simulink model "Reactor_PDE_R2013a"  (R2013a)
settings: Solver=ode45  StartTime=0.0  StopTime=double(Tsim)  FixedStep=double(grampc.param.dt)  RelTol=1e-3
values from neighbouring files (symbols this model uses):
  grampc = grampc_update_struct_grampc(grampc,user)    [initData.m]    (also in startMPC.m = CmexFiles.grampc_setparam_Cmex(grampc,'x0',vec.x(:,i)))
settings Model: Creator=kaepernick  LastModifiedBy=koy47
settings OptimizationCC: ExpressionDepthLimit=2147483647
settings DebuggingCC: FrameProcessingCompatibilityMsg=error
settings GRTTargetCC: CodeReplacementLibrary=C89/C90 (ANSI)

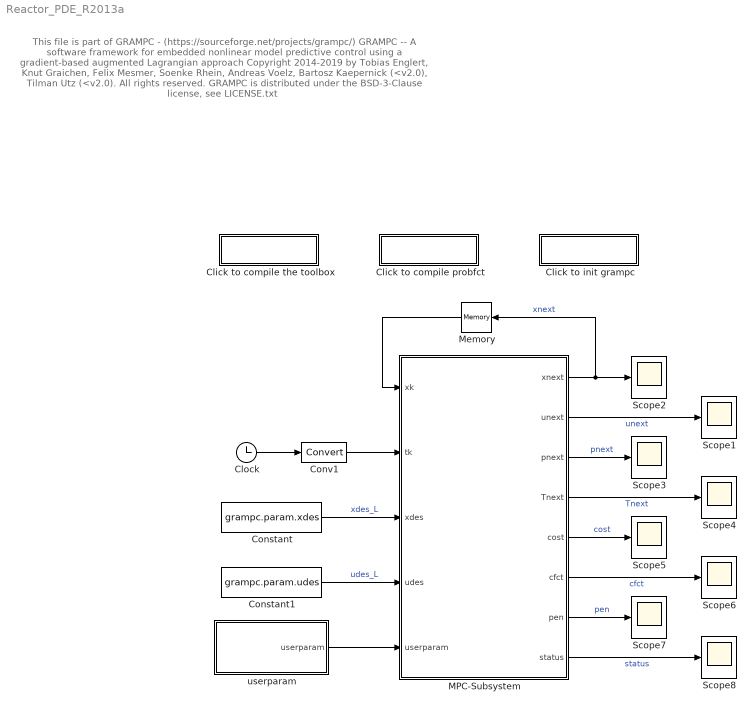
== system Reactor_PDE_R2013a ==
  note: This file is part of GRAMPC - (https://sourceforge.net/projects/grampc/)
      |
      | GRAMPC -- A software framework for embedded nonlinear model predictive
      | control using a gradient-based augmented Lagrangian approach
      |
      | Copyright 2014-2019 by Tobias Englert, Knut Graichen, Felix Mesmer,
      | Soenke Rhein, Andreas Voelz, Bartosz Kaepernick (<v2.0), Tilman Utz (<v2.0).
      | All rights reserved.
      |
      | GRAMPC is distributed under the BSD-3-Clause license, see LICENSE.txt
  Click to compile probfct : Subsystem
      settings: OpenFcn=|
      | cd(fileparts(which(gcs)))
      | grampc_path = '../../';
      | addpath([grampc_path 'matlab/mfiles']);
      | grampc_make_probfct(grampc_path,'probfct_REACTOR_PDE.c','clean');
  Click to compile the toolbox : Subsystem
      settings: OpenFcn=|
      | cd(fileparts(which(gcs)))
      | curdir = cd;
      | cd('../../matlab')
      | make clean
      | cd(curdir)
  Click to init grampc : Subsystem
      settings: OpenFcn=|
      | cd(fileparts(which(gcs)))
      | grampc_path = '../../';
      | addpath([grampc_path 'matlab/mfiles']);
      | [grampc,Tsim,grampc_sdata] = initData;
  Clock : Clock
  Constant : Constant  Value=grampc.param.xdes
  Constant1 : Constant  Value=grampc.param.udes
  Conv1 : DataTypeConversion
  MPC-Subsystem : Subsystem  TreatAsAtomicUnit=on  SystemSampleTime=double(grampc.param.dt)
  Memory : Memory  X0=grampc.param.x0
  Scope{1..8} (8 alike) : Scope
      Scope1 settings: TimeRange=auto  MaxDataPoints=5000  SaveToWorkspace=off  YMin=-2.5  YMax=2.5  SampleTime=-1
      Scope2 settings: TimeRange=auto  MaxDataPoints=5000  SaveToWorkspace=off  SaveName=ScopeData2  YMin=0.66111  YMax=2.14906  SampleTime=-1
      Scope3 settings: TimeRange=auto  MaxDataPoints=5000  SaveToWorkspace=off  SaveName=ScopeData3  YMin=-1.00000  YMax=1.00000  SampleTime=-1
      Scope4 settings: TimeRange=auto  MaxDataPoints=5000  SaveToWorkspace=off  SaveName=ScopeData4  YMin=0.5  YMax=2.5  SampleTime=-1
      Scope5 settings: TimeRange=auto  MaxDataPoints=5000  SaveToWorkspace=off  SaveName=ScopeData5  YMin=-0.1279  YMax=0.27397  SampleTime=-1
      Scope6 settings: TimeRange=auto  MaxDataPoints=5000  SaveToWorkspace=off  SaveName=ScopeData6  YMin=-0.15393  YMax=1.38537  SampleTime=-1
      Scope7 settings: TimeRange=auto  MaxDataPoints=5000  SaveToWorkspace=off  SaveName=ScopeData7  YMin=-28.95426  YMax=270.07514  SampleTime=-1
      Scope8 settings: TimeRange=auto  MaxDataPoints=5000  SaveToWorkspace=off  SaveName=ScopeData8  YMin=-36.00000  YMax=324.00000  SampleTime=-1
  userparam : Subsystem
  wires:
  MPC-Subsystem/6(cfct) -> Scope6/1  "cfct"
  MPC-Subsystem/3(pnext) -> Scope3/1  "pnext"
  MPC-Subsystem/8(status) -> Scope8/1  "status"
  MPC-Subsystem/4(Tnext) -> Scope4/1  "Tnext"
  MPC-Subsystem/1(xnext) -> Memory/1, Scope2/1  "xnext"
  Constant1/1 -> MPC-Subsystem/4(udes)  "udes_L"
  MPC-Subsystem/7(pen) -> Scope7/1  "pen"
  Constant/1 -> MPC-Subsystem/3(xdes)  "xdes_L"
  MPC-Subsystem/5(cost) -> Scope5/1  "cost"
  MPC-Subsystem/2(unext) -> Scope1/1  "unext"
  Conv1/1 -> MPC-Subsystem/2(tk)
  Clock/1 -> Conv1/1
  Memory/1 -> MPC-Subsystem/1(xk)
  userparam/1(userparam) -> MPC-Subsystem/5(userparam)

== system Reactor_PDE_R2013a/Click to compile probfct ==

== system Reactor_PDE_R2013a/Click to compile the toolbox ==

== system Reactor_PDE_R2013a/Click to init grampc ==

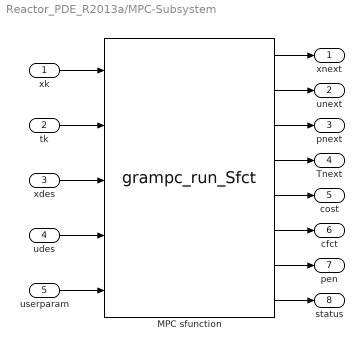
== system Reactor_PDE_R2013a/MPC-Subsystem ==
  xk : Inport
  tk : Inport  Port=2
  xdes : Inport  Port=3
  udes : Inport  Port=4
  userparam : Inport  Port=5
  MPC sfunction : S-Function  FunctionName=grampc_run_Sfct  Parameters=grampc_sdata.intoptidx grampc_sdata.intopt grampc_sdata.numoptidx grampc_sdata.numopt grampc_sdata.numparamidx grampc_sdata.numparam  SFunctionDeploymentMode=off  EnableBusSupport=off
      mask Display:
      | port_label('input',1,'x0')
      | port_label('input',2,'t0')
      | port_label('input',3,'xdes')
      | port_label('input',4,'udes')
      | port_label('input',5,'userparam')
      | 
      | port_label('output',1,'xnext')
      | port_label('output',2,'unext')
      | port_label('output',3,'pnext')
      | port_label('output',4,'Tnext')
      | port_label('output',5,'cost')
      | port_label('output',6,'||cfct||')
      | port_label('output',7,'||pen||')
      | port_label('output',8,'status')
      | 
      | disp('GRAMPC')
  xnext : Outport
  unext : Outport  Port=2
  pnext : Outport  Port=3
  Tnext : Outport  Port=4
  cost : Outport  Port=5
  cfct : Outport  Port=6
  pen : Outport  Port=7
  status : Outport  Port=8
  wires:
  xk/1 -> MPC sfunction/1
  MPC sfunction/1 -> xnext/1
  MPC sfunction/8 -> status/1
  MPC sfunction/7 -> pen/1
  xdes/1 -> MPC sfunction/3
  MPC sfunction/6 -> cfct/1
  udes/1 -> MPC sfunction/4
  MPC sfunction/5 -> cost/1
  MPC sfunction/3 -> pnext/1
  MPC sfunction/4 -> Tnext/1
  MPC sfunction/2 -> unext/1
  tk/1 -> MPC sfunction/2
  userparam/1 -> MPC sfunction/5

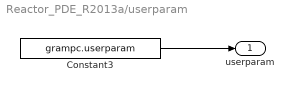
== system Reactor_PDE_R2013a/userparam ==
  Constant3 : Constant  Value=grampc.userparam
  userparam : Outport
  wires:
  Constant3/1 -> userparam/1
